simulink model "solar_panel_ratcking"  (R2021a)
settings: Solver=VariableStepAuto  StartTime=0.0  StopTime=10.0  RelTol=1e-3
values from neighbouring files (symbols this model uses):
  J = 5    [data_motor2.m]
undefined symbols (not defined in the file or in its folder): Kd
settings Model: Creator=Davie  LastModifiedBy=Davie

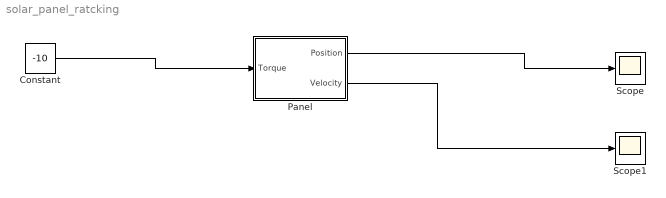
== system solar_panel_ratcking ==
  Constant : Constant  Value=-10
  Panel : Subsystem
  Scope : Scope
  Scope1 : Scope
  wires:
  Constant/1 -> Panel/1(Torque)
  Panel/1(Position) -> Scope/1
  Panel/2(Velocity) -> Scope1/1

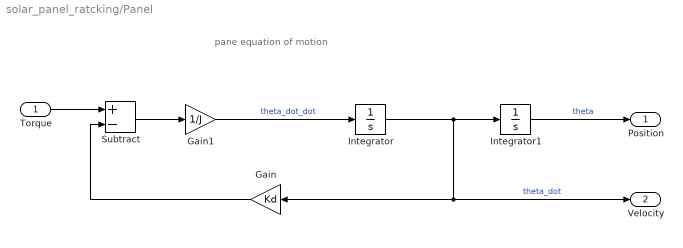
== system solar_panel_ratcking/Panel ==
  note: pane equation of motion
  Torque : Inport
  Gain : Gain  Gain=Kd
  Gain1 : Gain  Gain=1/J
  Integrator : Integrator
  Integrator1 : Integrator
  Subtract : Sum  Inputs=+-
  Position : Outport
  Velocity : Outport  Port=2
  wires:
  Integrator/1 -> Velocity/1, Gain/1, Integrator1/1  "theta_dot"
  Gain/1 -> Subtract/2
  Subtract/1 -> Gain1/1
  Gain1/1 -> Integrator/1  "theta_dot_dot"
  Integrator1/1 -> Position/1  "theta"
  Torque/1 -> Subtract/1
